simulink model "motor_dynamics"  (R2020a)
settings: Solver=VariableStepAuto  StartTime=0.0  StopTime=10.0  RelTol=1e-3
undefined symbols (not defined in the file): b, J, K, L, Res
settings Model: Creator=daixingze  LastModifiedBy=daixingze

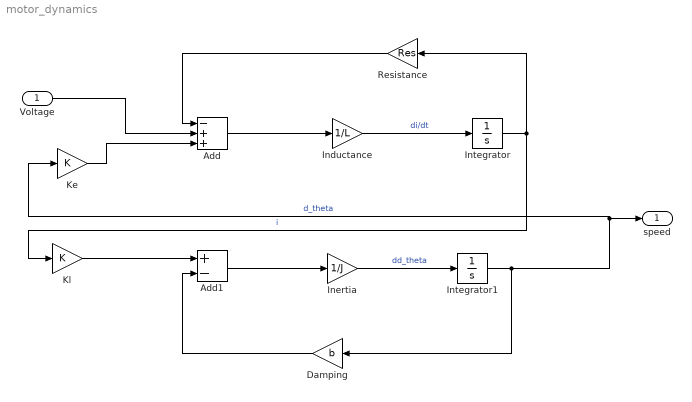
== system motor_dynamics ==
  Voltage : Inport
  Add : Sum  Inputs=-++
  Add1 : Sum  Inputs=+-
  Damping : Gain  Gain=b
  Inductance : Gain  Gain=1/L
  Inertia : Gain  Gain=1/J
  Integrator : Integrator
  Integrator1 : Integrator
  Ke : Gain  Gain=K
  Kl : Gain  Gain=K
  Resistance : Gain  Gain=Res
  speed : Outport
  wires:
  Voltage/1 -> Add/2
  Ke/1 -> Add/3
  Add/1 -> Inductance/1
  Inductance/1 -> Integrator/1  "di/dt"
  Integrator/1 -> Kl/1, Resistance/1  "i"
  Resistance/1 -> Add/1
  Kl/1 -> Add1/1
  Add1/1 -> Inertia/1
  Inertia/1 -> Integrator1/1  "dd_theta"
  Integrator1/1 -> Ke/1, speed/1, Damping/1  "d_theta"
  Damping/1 -> Add1/2
